simulink model "SingleTrack"  (R2019b)
settings: Solver=ode1  StartTime=0  StopTime=250  FixedStep=1.0000000000000000e-003  RelTol=1e-3
InitFcn:
  | sampleTime = str2double(get_param(bdroot, 'FixedStep'));
undefined symbols (not defined in the file or in its folder): AccPedalPos, BrakePedalPos, BrakeSwitch, DiscIntNeverNeededParam, DYNA4, EngSpd, IgnitionSwitch, InitialGear, InitialSpeed, IntendedEngTrq, LeftIndicator, MainBrakePress, MaxGear, MDL, MinGear, RefAcc, RefLane, RefLatPos, RefPath, RefPathCurv, RefSpd, RefSpdPreview, RefSpdRetrospect, RightIndicator, SteeringWheelAng, SteeringWheelTrq, UserDefinedRefValue, vm_const
libraries: UtilitiesLibrary x31, simulink x18, WheelSystemModules x13, LongitudinalControllerModules x13, LateralControllerModules x7, AnimationBusselectorModules x5, EnvironmentModules x5, BasicEngineControlModules x5, MiscellaneousControlModules x5, Animation3Modules x4, AuxiliariesModules x4, ReducedTireModules x4
(part 6 of 32)

== system SingleTrack/Vehicle/Engine ==
  fromCTRL : Inport
  fromEnvironment : Inport  Port=2
  fromChassis : Inport  Port=3
  fromDrivetrain : Inport  Port=4
  fromElectricalSystem : Inport  Port=5
  DYNA4 Trace Marker : UtilitiesLibrary/DYNA4 Trace Marker  Tag=DYNA4_TRACE_MARKER  SettingType=Standard  PrefixModelBlockID=on  PrefixRootSignalName=off  NamePattern='$(modelBlockID).$(rootSignalName)'
  DynaComponentInfo : Subsystem  Tag=DynaComponentInfo
      mask init:
      | data= get_param(gcb, 'UserData');
      settings: OpenFcn=DYNA4.ModelHandling.Component.ShowEditComponentInformationDialog(gcb);
      mask Display: disp(['Type = ', data.type, '\nGroup = ', data.group, '\nName = ', data.name ])
  EngineControlUnit : Subsystem  Tag=COMPONENT_ENGINE
  EngineOutputs : Subsystem  Tag=TESIS DYNAware Interface Block  mask{NeedsUpdate=off, SignalInfo=|}
      mask SignalInfo=|
      | {
      |   "Version": "4.6",
      |   "MuxedOutputBusName": "Engine",
      |   "MuxedInputBusName": "",
      |   "MuxedInputSelected": false,
      |   "MuxedOutputSelected": true,
      |   "SignalData": [
      |     {
      |       "initialValue": "0.0",
      |       "name": "EnginePhysics",
      |       "comment": "",
      |       "minString": "",
      |       "maxString": "",
      |       "width": -1,
      |       "dataType": 0,
      |       "signalType": 1,
      |       "createSignal": false,
      |       "outputName": "EnginePhysics",
      |       "generateSignalAccessBlock": false,
      |       "accessId": "$(parentId).$(blockName).$(outputName)"
      |     },
      |     {
      |       "initialValue": "0.0",
      |       "name": "EngineControlUnit",
      |       "comment": "",
      |       "minString": "",
      |       "maxString": "",
      |       "width": -1,
      |       "dataType": 0,
      |       "signalType": 1,
      |       "createSignal": false,
      |       "outputName": "EngineControlUnit",
      |       "generateSignalAccessBlock": false,
      |       "accessId": "$(parentId).$(blockName).$(outputName)"
      |     }
      |   ]
      | }
      mask prompts: NeedsUpdate "Specify, if subsystem content needs to be updated"; SignalInfo "Signal Info (json)"
      mask help: DYNA4 Interface Block Version 4.6
      mask init:
      | blockName = get_param(gcbh, 'Name');
      | parentId = DYNA4.ModelHandling.AccessID.getFromHierarchy(gcbh);
      | TD.InterfaceBlock.ModelCallbacks.GenerateContent(gcb);
      settings: DeleteFcn=TD.InterfaceBlock.ModelCallbacks.CloseGUI( gcbh );  NameChangeFcn=TD.InterfaceBlock.ModelCallbacks.BlockRenamedHandler(gcbh);  OpenFcn=TD.InterfaceBlock.ModelCallbacks.OpenGUI( gcbh );  CloseFcn=TD.InterfaceBlock.ModelCallbacks.CloseGUI( gcbh );
      mask Display:
      | image('InterfaceBlock.png','center');
      | port_label('input',1, 'EnginePhysics');
      | port_label('input',2, 'EngineControlUnit');
      | port_label('output',1, 'Engine');
  EnginePhysics : Subsystem  Tag=COMPONENT_ENGINE
  Engine : Outport  VectorParamsAs1DForOutWhenUnconnected=off
  wires:
  fromChassis/1 -> EnginePhysics/4(fromChassis), EngineControlUnit/4(fromChassis)
  EngineControlUnit/1(EngineControlUnit) -> EngineOutputs/2(EngineControlUnit___UNIQUE_1), EnginePhysics/1(fromEngineControlUnit)
  fromCTRL/1 -> EnginePhysics/2(fromCTRL), EngineControlUnit/2(fromCTRL)
  fromElectricalSystem/1 -> EnginePhysics/6(fromElectricalSystem), EngineControlUnit/6(fromElectricalSystem)
  fromEnvironment/1 -> EnginePhysics/3(fromEnvironment), EngineControlUnit/3(fromEnvironment)
  EngineOutputs/1(Engine___UNIQUE_1) -> Engine/1, DYNA4 Trace Marker/1
  fromDrivetrain/1 -> EnginePhysics/5(fromDrivetrain), EngineControlUnit/5(fromDrivetrain)
  EnginePhysics/1(EnginePhysics) -> EngineOutputs/1(EnginePhysics___UNIQUE_1), EngineControlUnit/1(fromEnginePhysics)

== system SingleTrack/Vehicle/VehicleOutput ==
  Auxiliaries___UNIQUE_1 : Inport  Description=|
      | <name>Auxiliaries</name>
      | <comment></comment>
  BrakeSystem___UNIQUE_1 : Inport  Description=|  Port=2
      | <name>BrakeSystem</name>
      | <comment></comment>
  Chassis___UNIQUE_1 : Inport  Description=|  Port=3
      | <name>Chassis</name>
      | <comment></comment>
  Drivetrain___UNIQUE_1 : Inport  Description=|  Port=4
      | <name>Drivetrain</name>
      | <comment></comment>
  ElectricalSystem___UNIQUE_1 : Inport  Description=|  Port=5
      | <name>ElectricalSystem</name>
      | <comment></comment>
  Engine___UNIQUE_1 : Inport  Description=|  Port=6
      | <name>Engine</name>
      | <comment></comment>
  WheelSystem___UNIQUE_1 : Inport  Description=|  Port=7
      | <name>WheelSystem</name>
      | <comment></comment>
  CoolingSystem___UNIQUE_1 : Inport  Description=|  Port=8
      | <name>CoolingSystem</name>
      | <comment></comment>
  VehicleRoadInfo___UNIQUE_1 : Inport  Description=|  Port=9
      | <name>VehicleRoadInfo</name>
      | <comment></comment>
  VehicleDriverInfo___UNIQUE_1 : Inport  Description=|  Port=10
      | <name>VehicleDriverInfo</name>
      | <comment></comment>
  __TDO__Vehicle : BusCreator  Inputs=10
  Vehicle___UNIQUE_1 : Outport  Description=|  VectorParamsAs1DForOutWhenUnconnected=off
      | <name>Auxiliaries</name>
      | <comment></comment>
  wires:
  __TDO__Vehicle/1 -> Vehicle___UNIQUE_1/1  "Vehicle"
  VehicleDriverInfo___UNIQUE_1/1 -> __TDO__Vehicle/10  "VehicleDriverInfo"
  VehicleRoadInfo___UNIQUE_1/1 -> __TDO__Vehicle/9  "VehicleRoadInfo"
  CoolingSystem___UNIQUE_1/1 -> __TDO__Vehicle/8  "CoolingSystem"
  WheelSystem___UNIQUE_1/1 -> __TDO__Vehicle/7  "WheelSystem"
  Engine___UNIQUE_1/1 -> __TDO__Vehicle/6  "Engine"
  ElectricalSystem___UNIQUE_1/1 -> __TDO__Vehicle/5  "ElectricalSystem"
  Drivetrain___UNIQUE_1/1 -> __TDO__Vehicle/4  "Drivetrain"
  Chassis___UNIQUE_1/1 -> __TDO__Vehicle/3  "Chassis"
  BrakeSystem___UNIQUE_1/1 -> __TDO__Vehicle/2  "BrakeSystem"
  Auxiliaries___UNIQUE_1/1 -> __TDO__Vehicle/1  "Auxiliaries"

== system SingleTrack/Vehicle/VehicleRoadInfo ==
  fromCTRL : Inport
  fromChassis : Inport  Port=2
  AdditionalRoadElevationAndRoadSlopes : Subsystem
  Demux : Demux  Outputs=3
  Demux1 : Demux  Outputs=2
  Demux2 : Demux  Outputs=2
  DynaComponentInfo : Subsystem  Tag=DynaComponentInfo
      mask init:
      | data = get_param(gcb, 'UserData');
      settings: OpenFcn=DYNA4.ModelHandling.Component.ShowEditComponentInformationDialog(gcb);
      mask Display: disp(['Type = ', data.type, '\nGroup = ', data.group, '\nName = ', data.name ])
  InputFromCTRL : Subsystem  Tag=TESIS DYNAware Interface Block  mask{NeedsUpdate=off, SignalInfo=|}
      mask SignalInfo=|
      | {
      |   "Version": "4.6",
      |   "MuxedOutputBusName": "output",
      |   "MuxedInputBusName": "fromCTRL",
      |   "MuxedInputSelected": true,
      |   "MuxedOutputSelected": false,
      |   "SignalData": [
      |     {
      |       "initialValue": "0.0",
      |       "name": "CTRL.AdditionalRoadElevation.FrontLeftAddRoadElev[m]",
      |       "comment": "",
      |       "minString": "",
      |       "maxString": "",
      |       "width": 1,
      |       "dataType": 0,
      |       "signalType": 0,
      |       "createSignal": false,
      |       "outputName": "FrontLeftAddRoadElev[m]",
      |       "generateSignalAccessBlock": false,
      |       "accessId": "$(parentId).$(blockName).$(outputName)"
      |     },
      |     {
      |       "initialValue": "0.0",
      |       "name": "CTRL.AdditionalRoadElevation.FrontRightAddRoadElev[m]",
      |       "comment": "",
      |       "minString": "",
      |       "maxString": "",
      |       "width": 1,
      |       "dataType": 0,
      |       "signalType": 0,
      |       "createSignal": false,
      |       "outputName": "FrontRightAddRoadElev[m]",
      |       "generateSignalAccessBlock": false,
      |       "accessId": "$(parentId).$(blockName).$(outputName)"
      |     },
      |     {
      |       "initialValue": "0.0",
      |       "name": "CTRL.AdditionalRoadElevation.AddLongRoadSlope[-]",
      |       "comment": "",
      |       "minString": "",
      |       "maxString": "",
      |       "width": 1,
      |       "dataType": 0,
      |       "signalType": 0,
      |       "createSignal": false,
      |       "outputName": "AddLongRoadSlope[-]",
      |       "generateSignalAccessBlock": false,
      |       "accessId": "$(parentId).$(blockName).$(outputName)"
      |     },
      |     {
      |       "initialValue": "0.0",
      |       "name": "CTRL.AdditionalRoadElevation.AddLatRoadSlope[-]",
      |       "comment": "",
      |       "minString": "",
      |       "maxString": "",
      |       "width": 1,
      |       "dataType": 0,
      |       "signalType": 0,
      |       "createSignal": false,
      |       "outputName": "AddLatRoadSlope[-]",
      |       "generateSignalAccessBlock": false,
      |       "accessId": "$(parentId).$(blockName).$(outputName)"
      |     },
      |     {
      |       "initialValue": "0.0",
      |       "name": "CTRL.AdditionalRoadElevation.LocalRoadSysSwitch[0;1]",
      |       "comment": "",
      |       "minString": "",
      |       "maxString": "",
      |       "width": 1,
      |       "dataType": 0,
      |       "signalType": 0,
      |       "createSignal": false,
      |       "outputName": "LocalRoadSysSwitch[0;1]",
      |       "generateSignalAccessBlock": false,
      |       "accessId": "$(parentId).$(blockName).$(outputName)"
      |     }
      |   ]
      | }
      mask prompts: NeedsUpdate "Specify, if subsystem content needs to be updated"; SignalInfo "Signal Info (json)"
      mask help: DYNA4 Interface Block Version 4.6
      mask init:
      | blockName = get_param(gcbh, 'Name');
      | parentId = DYNA4.ModelHandling.AccessID.getFromHierarchy(gcbh);
      | TD.InterfaceBlock.ModelCallbacks.GenerateContent(gcb);
      settings: DeleteFcn=TD.InterfaceBlock.ModelCallbacks.CloseGUI( gcbh );  NameChangeFcn=TD.InterfaceBlock.ModelCallbacks.BlockRenamedHandler(gcbh);  OpenFcn=TD.InterfaceBlock.ModelCallbacks.OpenGUI( gcbh );  CloseFcn=TD.InterfaceBlock.ModelCallbacks.CloseGUI( gcbh );
      mask Display:
      | image('InterfaceBlock.png','center');
      | port_label('input',1, 'fromCTRL');
      | port_label('output',1, 'FrontLeftAddRoadElev[m]');
      | port_label('output',2, 'FrontRightAddRoadElev[m]');
      | port_label('output',3, 'AddLongRoadSlope[-]');
      | port_label('output',4, 'AddLatRoadSlope[-]');
      | port_label('output',5, 'LocalRoadSysSwitch[0;1]');
  InputFromChassis : Subsystem  Tag=TESIS DYNAware Interface Block  mask{NeedsUpdate=off, SignalInfo=|}
      mask SignalInfo=|
      | {
      |   "Version": "4.6",
      |   "MuxedOutputBusName": "output",
      |   "MuxedInputBusName": "fromChassis",
      |   "MuxedInputSelected": true,
      |   "MuxedOutputSelected": false,
      |   "SignalData": [
      |     {
      |       "initialValue": "0.0",
      |       "name": "VehicleBody.Pos(WorldSys)[m]",
      |       "comment": "",
      |       "minString": "",
      |       "maxString": "",
      |       "width": 3,
      |       "dataType": 0,
      |       "signalType": 0,
      |       "createSignal": false,
      |       "outputName": "Pos(WorldSys)[m]",
      |       "generateSignalAccessBlock": false,
      |       "accessId": "$(parentId).$(blockName).$(outputName)"
      |     },
      |     {
      |       "initialValue": "0.0",
      |       "name": "VehicleBody.YawAng[rad]",
      |       "comment": "",
      |       "minString": "",
      |       "maxString": "",
      |       "width": 1,
      |       "dataType": 0,
      |       "signalType": 0,
      |       "createSignal": false,
      |       "outputName": "YawAng[rad]",
      |       "generateSignalAccessBlock": false,
      |       "accessId": "$(parentId).$(blockName).$(outputName)"
      |     }
      |   ]
      | }
      mask prompts: NeedsUpdate "Specify, if subsystem content needs to be updated"; SignalInfo "Signal Info (json)"
      mask help: DYNA4 Interface Block Version 4.6
      mask init:
      | blockName = get_param(gcbh, 'Name');
      | parentId = DYNA4.ModelHandling.AccessID.getFromHierarchy(gcbh);
      | TD.InterfaceBlock.ModelCallbacks.GenerateContent(gcb);
      settings: DeleteFcn=TD.InterfaceBlock.ModelCallbacks.CloseGUI( gcbh );  NameChangeFcn=TD.InterfaceBlock.ModelCallbacks.BlockRenamedHandler(gcbh);  OpenFcn=TD.InterfaceBlock.ModelCallbacks.OpenGUI( gcbh );  CloseFcn=TD.InterfaceBlock.ModelCallbacks.CloseGUI( gcbh );
      mask Display:
      | image('InterfaceBlock.png','center');
      | port_label('input',1, 'fromChassis');
      | port_label('output',1, 'Pos(WorldSys)[m]');
      | port_label('output',2, 'YawAng[rad]');
  Road Information : RoadModules/Road Information  RoadQueryType=X, Y (WorldSystem)  RoadQueryNumber=1  ODR_ALL_FLAGS=off  ODR_TRACKID=on  ODR_LANEID=on  ODR_XY=off  ODR_Z=on  ODR_S_ROAD=on  ODR_Q_ROAD=on  ODR_Q_PATH=off  ODR_QMINMAX_ROAD=off  ODR_QMINMAX_PATH=off  ODR_XY_REF=off  ODR_GEO_COORDINATES=off  ODR_ANGLE_ROAD=on  ODR_ANGLE_PATH=off  ODR_CURVATURE_ROAD=on  ODR_CURVATURE_PATH=on  ODR_TXTY_ROAD=on  ODR_PITCHROLL_ROAD=off  ODR_SQSLOPE_ROAD=on  ODR_MATERIAL=on  ODR_LATERAL_INFO=off  ODR_NEXT_DRIVEABLE_LANEID=off  ODR_ROAD_MARKS=off  ODR_VMAX=off  ODR_ROAD_SIGNS=off  ODR_ROUTE=off  ODR_JUNCTION=off  ODR_ROAD_LANE_LIST=off  ODR_LENGTH_CLOSED=on  EnableSeparateRoute=off  RoutePointsTrackIDs=MDL.Traffic.TrafficObjects.Traffic.Route{1}.RoutePointsTrackIDs.v  RoutePointsSCoordOnTrack=MDL.Traffic.TrafficObjects.Traffic.Route{1}.RoutePointsSCoordOnTrack.v  sample_time=-1
  Selector1 : Selector  InputPortWidth=3  IndexOptions=Index vector (dialog)  Indices=[1 2]  OutputSizes=1
  Selector2 : Selector  InputPortWidth=6  IndexOptions=Index vector (dialog)  Indices=[1 2]  OutputSizes=1
  Sum : Sum  Inputs=|++
  Sum1 : Sum  Inputs=|++
  Sum3 : Sum  Inputs=|++
  Terminator : Terminator
  TraceMarker : UtilitiesLibrary/DYNA4 Trace Marker  Tag=DYNA4_TRACE_MARKER  SettingType=Standard  PrefixModelBlockID=on  PrefixRootSignalName=off  NamePattern='$(modelBlockID).$(rootSignalName)'
  VehicleRoadInfoOutput : Subsystem  Tag=TESIS DYNAware Interface Block  mask{NeedsUpdate=off, SignalInfo=|}
      mask SignalInfo=|
      | {
      |   "Version": "4.6",
      |   "MuxedOutputBusName": "VehicleRoadInfo",
      |   "MuxedInputBusName": "input",
      |   "MuxedInputSelected": false,
      |   "MuxedOutputSelected": true,
      |   "SignalData": [
      |     {
      |       "initialValue": "0.0",
      |       "name": "TrackID[-]",
      |       "comment": "",
      |       "minString": "",
      |       "maxString": "",
      |       "width": 1,
      |       "dataType": 0,
      |       "signalType": 0,
      |       "createSignal": false,
      |       "outputName": "TrackID[-]",
      |       "generateSignalAccessBlock": false,
      |       "accessId": "$(parentId).$(blockName).$(outputName)"
      |     },
      |     {
      |       "initialValue": "0.0",
      |       "name": "LaneID[-]",
      |       "comment": "",
      |       "minString": "",
      |       "maxString": "",
      |       "width": 1,
      |       "dataType": 0,
      |       "signalType": 0,
      |       "createSignal": false,
      |       "outputName": "LaneID[-]",
      |       "generateSignalAccessBlock": false,
      |       "accessId": "$(parentId).$(blockName).$(outputName)"
      |     },
      |     {
      |       "initialValue": "0.0",
      |       "name": "RoadZ[m]",
      |       "comment": "",
      |       "minString": "",
      |       "maxString": "",
      |       "width": 1,
      |       "dataType": 0,
      |       "signalType": 0,
      |       "createSignal": false,
      |       "outputName": "RoadZ[m]",
      |       "generateSignalAccessBlock": false,
      |       "accessId": "$(parentId).$(blockName).$(outputName)"
      |     },
      |     {
      |       "initialValue": "0.0",
      |       "name": "RoadS[m]",
      |       "comment": "",
      |       "minString": "",
      |       "maxString": "",
      |       "width": 1,
      |       "dataType": 0,
      |       "signalType": 0,
      |       "createSignal": false,
      |       "outputName": "RoadS[m]",
      |       "generateSignalAccessBlock": false,
      |       "accessId": "$(parentId).$(blockName).$(outputName)"
      |     },
      |     {
      |       "initialValue": "0.0",
      |       "name": "RoadQ[m]",
      |       "comment": "",
      |       "minString": "",
      |       "maxString": "",
      |       "width": 1,
      |       "dataType": 0,
      |       "signalType": 0,
      |       "createSignal": false,
      |       "outputName": "RoadQ[m]",
      |       "generateSignalAccessBlock": false,
      |       "accessId": "$(parentId).$(blockName).$(outputName)"
      |     },
      |     {
      |       "initialValue": "0.0",
      |       "name": "RoadAngle[rad]",
      |       "comment": "",
      |       "minString": "",
      |       "maxString": "",
      |       "width": 1,
      |       "dataType": 0,
      |       "signalType": 0,
      |       "createSignal": false,
      |       "outputName": "RoadAngle[rad]",
      |       "generateSignalAccessBlock": false,
      |       "accessId": "$(parentId).$(blockName).$(outputName)"
      |     },
      |     {
      |       "initialValue": "0.0",
      |       "name": "RoadCurvature[1/m]",
      |       "comment": "",
      |       "minString": "",
      |       "maxString": "",
      |       "width": 1,
      |       "dataType": 0,
      |       "signalType": 0,
      |       "createSignal": false,
      |       "outputName": "RoadCurvature[1/m]",
      |       "generateSignalAccessBlock": false,
      |       "accessId": "$(parentId).$(blockName).$(outputName)"
      |     },
      |     {
      |       "initialValue": "0.0",
      |       "name": "LaneCurvature[1/m]",
      |       "comment": "",
      |       "minString": "",
      |       "maxString": "",
      |       "width": 1,
      |       "dataType": 0,
      |       "signalType": 0,
      |       "createSignal": false,
      |       "outputName": "LaneCurvature[1/m]",
      |       "generateSignalAccessBlock": false,
      |       "accessId": "$(parentId).$(blockName).$(outputName)"
      |     },
      |     {
      |       "initialValue": "0.0",
      |       "name": "RoadTangentXY[-]",
      |       "comment": "",
      |       "minString": "",
      |       "maxString": "",
      |       "width": 2,
      |       "dataType": 0,
      |       "signalType": 0,
      |       "createSignal": false,
      |       "outputName": "RoadTangentXY[-]",
      |       "generateSignalAccessBlock": false,
      |       "accessId": "$(parentId).$(blockName).$(outputName)"
      |     },
      |     {
      |       "initialValue": "0.0",
      |       "name": "RoadSlopeLong[-]",
      |       "comment": "",
      |       "minString": "",
      |       "maxString": "",
      |       "width": 1,
      |       "dataType": 0,
      |       "signalType": 0,
      |       "createSignal": false,
      |       "outputName": "RoadSlopeLong[-]",
      |       "generateSignalAccessBlock": false,
      |       "accessId": "$(parentId).$(blockName).$(outputName)"
      |     },
      |     {
      |       "initialValue": "0.0",
      |       "name": "RoadSlopeLat[-]",
      |       "comment": "",
      |       "minString": "",
      |       "maxString": "",
      |       "width": 1,
      |       "dataType": 0,
      |       "signalType": 0,
      |       "createSignal": false,
      |       "outputName": "RoadSlopeLat[-]",
      |       "generateSignalAccessBlock": false,
      |       "accessId": "$(parentId).$(blockName).$(outputName)"
      |     },
      |     {
      |       "initialValue": "0.0",
      |       "name": "RoadFriction[-]",
      |       "comment": "",
      |       "minString": "",
      |       "maxString": "",
      |       "width": 1,
      |       "dataType": 0,
      |       "signalType": 0,
      |       "createSignal": false,
      |       "outputName": "RoadFriction[-]",
      |       "generateSignalAccessBlock": false,
      |       "accessId": "$(parentId).$(blockName).$(outputName)"
      |     },
      |     {
      |       "initialValue": "0.0",
      |       "name": "RoadSurfaceType[-]",
      |       "comment": "",
      |       "minString": "",
      |       "maxString": "",
      |       "width": 1,
      |       "dataType": 0,
      |       "signalType": 0,
      |       "createSignal": false,
      |       "outputName": "RoadSurfaceType[-]",
      |       "generateSignalAccessBlock": false,
      |       "accessId": "$(parentId).$(blockName).$(outputName)"
      |     },
      |     {
      |       "initialValue": "0.0",
      |       "name": "RoadRoughness[-]",
      |       "comment": "",
      |       "minString": "",
      |       "maxString": "",
      |       "width": 1,
      |       "dataType": 0,
      |       "signalType": 0,
      |       "createSignal": false,
      |       "outputName": "RoadRoughness[-]",
      |       "generateSignalAccessBlock": false,
      |       "accessId": "$(parentId).$(blockName).$(outputName)"
      |     },
      |     {
      |       "initialValue": "0.0",
      |       "name": "RouteLength[m]",
      |       "comment": "",
      |       "minString": "",
      |       "maxString": "",
      |       "width": 1,
      |       "dataType": 0,
      |       "signalType": 0,
      |       "createSignal": false,
      |       "outputName": "RouteLength[m]",
      |       "generateSignalAccessBlock": false,
      |       "accessId": "$(parentId).$(blockName).$(outputName)"
      |     },
      |     {
      |       "initialValue": "0.0",
      |       "name": "RouteClosed[-]",
      |       "comment": "",
      |       "minString": "",
      |       "maxString": "",
      |       "width": 1,
      |       "dataType": 0,
      |       "signalType": 0,
      |       "createSignal": false,
      |       "outputName": "RouteClosed[-]",
      |       "generateSignalAccessBlock": false,
      |       "accessId": "$(parentId).$(blockName).$(outputName)"
      |     }
      |   ]
      | }
      mask prompts: NeedsUpdate "Specify, if subsystem content needs to be updated"; SignalInfo "Signal Info (json)"
      mask help: DYNA4 Interface Block Version 4.6
      mask init:
      | blockName = get_param(gcbh, 'Name');
      | parentId = DYNA4.ModelHandling.AccessID.getFromHierarchy(gcbh);
      | TD.InterfaceBlock.ModelCallbacks.GenerateContent(gcb);
      settings: DeleteFcn=TD.InterfaceBlock.ModelCallbacks.CloseGUI( gcbh );  NameChangeFcn=TD.InterfaceBlock.ModelCallbacks.BlockRenamedHandler(gcbh);  OpenFcn=TD.InterfaceBlock.ModelCallbacks.OpenGUI( gcbh );  CloseFcn=TD.InterfaceBlock.ModelCallbacks.CloseGUI( gcbh );
      mask Display:
      | image('InterfaceBlock.png','center');
      | port_label('input',1, 'TrackID[-]');
      | port_label('input',2, 'LaneID[-]');
      | port_label('input',3, 'RoadZ[m]');
      | port_label('input',4, 'RoadS[m]');
      | port_label('input',5, 'RoadQ[m]');
      | port_label('input',6, 'RoadAngle[rad]');
      | port_label('input',7, 'RoadCurvature[1/m]');
      | port_label('input',8, 'LaneCurvature[1/m]');
      | port_label('input',9, 'RoadTangentXY[-]');
      | port_label('input',10, 'RoadSlopeLong[-]');
      | port_label('input',11, 'RoadSlopeLat[-]');
      | port_label('input',12, 'RoadFriction[-]');
      | port_label('input',13, 'RoadSurfaceType[-]');
      | port_label('input',14, 'RoadRoughness[-]');
      | port_label('input',15, 'RouteLength[m]');
      | port_label('input',16, 'RouteClosed[-]');
      | port_label('output',1, 'VehicleRoadInfo');
  VehicleRoadInfo : Outport  VectorParamsAs1DForOutWhenUnconnected=off
  tag scope: VehicleRoadInfo=global
  wires:
  InputFromChassis/2(YawAng[rad]___UNIQUE_1) -> AdditionalRoadElevationAndRoadSlopes/1(YawAng[rad])
  InputFromChassis/1(Pos(WorldSys)[m]___UNIQUE_1) -> Selector1/1
  AdditionalRoadElevationAndRoadSlopes/3(AddLatRoadSlope[-]) -> Sum1/2
  AdditionalRoadElevationAndRoadSlopes/2(AddLongRoadSlope[-]) -> Sum/2
  AdditionalRoadElevationAndRoadSlopes/1(FrontAdditionalRoadElev[m]) -> Sum3/2
  InputFromCTRL/5(LocalRoadSysSwitch[0;1]___UNIQUE_1) -> AdditionalRoadElevationAndRoadSlopes/6(LocalRoadSysSwitch[0;1])
  InputFromCTRL/4(AddLatRoadSlope[-]___UNIQUE_1) -> AdditionalRoadElevationAndRoadSlopes/5(AddLatRoadSlopeIn[-])
  InputFromCTRL/3(AddLongRoadSlope[-]___UNIQUE_1) -> AdditionalRoadElevationAndRoadSlopes/4(AddLongRoadSlopeIn[-])
  InputFromCTRL/2(FrontRightAddRoadElev[m]___UNIQUE_1) -> AdditionalRoadElevationAndRoadSlopes/3(FrontRightAddRoadElev[m])
  InputFromCTRL/1(FrontLeftAddRoadElev[m]___UNIQUE_1) -> AdditionalRoadElevationAndRoadSlopes/2(FrontLeftAddRoadElev[m])
  Sum3/1 -> VehicleRoadInfoOutput/3(RoadZ[m]___UNIQUE_1)
  Road Information/3 -> Sum3/1
  Sum1/1 -> VehicleRoadInfoOutput/11(RoadSlopeLat[-]___UNIQUE_1)
  Demux1/2 -> Sum1/1
  Sum/1 -> VehicleRoadInfoOutput/10(RoadSlopeLong[-]___UNIQUE_1)
  Demux1/1 -> Sum/1
  fromCTRL/1 -> InputFromCTRL/1(fromCTRL)
  Road Information/12 -> Selector2/1
  Road Information/11 -> Demux/1
  Road Information/10 -> Demux1/1
  Road Information/9 -> VehicleRoadInfoOutput/9(RoadTangentXY[-]___UNIQUE_1)
  Road Information/8 -> VehicleRoadInfoOutput/8(LaneCurvature[1/m]___UNIQUE_1)
  Road Information/7 -> VehicleRoadInfoOutput/7(RoadCurvature[1/m]___UNIQUE_1)
  Selector2/1 -> Demux2/1
  Demux2/2 -> VehicleRoadInfoOutput/16(RouteClosed[-]___UNIQUE_1)
  Demux2/1 -> VehicleRoadInfoOutput/15(RouteLength[m]___UNIQUE_1)
  Demux/3 -> VehicleRoadInfoOutput/14(RoadRoughness[-]___UNIQUE_1)
  Demux/2 -> VehicleRoadInfoOutput/13(RoadSurfaceType[-]___UNIQUE_1)
  Demux/1 -> VehicleRoadInfoOutput/12(RoadFriction[-]___UNIQUE_1)
  Road Information/6 -> VehicleRoadInfoOutput/6(RoadAngle[rad]___UNIQUE_1)
  Road Information/5 -> VehicleRoadInfoOutput/5(RoadQ[m]___UNIQUE_1)
  Road Information/4 -> VehicleRoadInfoOutput/4(RoadS[m]___UNIQUE_1)
  Road Information/2 -> VehicleRoadInfoOutput/2(LaneID[-]___UNIQUE_1)
  Road Information/1 -> VehicleRoadInfoOutput/1(TrackID[-]___UNIQUE_1)
  Selector1/1 -> Road Information/2
  fromChassis/1 -> InputFromChassis/1(fromChassis)
  VehicleRoadInfoOutput/1(VehicleRoadInfo___UNIQUE_1) -> TraceMarker/1, [VehicleRoadInfo], VehicleRoadInfo/1
  [IRoadInterface] -> Road Information/1
  [VehicleRoadInfo] -> Terminator/1

== system SingleTrack/Vehicle/WheelSystem ==
  fromCTRL : Inport
  fromBrakeSystem : Inport  Port=2
  fromChassis : Inport  Port=3
  fromDrivetrain : Inport  Port=4
  DynaComponentInfo : Subsystem  Tag=DynaComponentInfo
      mask init:
      | data= get_param(gcb, 'UserData');
      settings: OpenFcn=DYNA4.ModelHandling.Component.ShowEditComponentInformationDialog(gcb);
      mask Display: disp(['Type = ', data.type, '\nGroup = ', data.group, '\nName = ', data.name])
  FrontLeftWheelSystem : Subsystem
  FrontRightWheelSystem : Subsystem
  RearLeftWheelSystem : Subsystem
  RearRightWheelSystem : Subsystem
  WheelSystemInputs : WheelSystemModules/WheelSystemInputs  SystemSampleTime=-1  Latency=0  AutoFrameSizeCalculation=off
  WheelSystemOutputs : Subsystem
  WheelSystem : Outport  VectorParamsAs1DForOutWhenUnconnected=off
  wires:
  WheelSystemInputs/12 -> RearLeftWheelSystem/4(fromBrakeSystem)
  RearRightWheelSystem/3(WheelStates) -> WheelSystemOutputs/12(RearRightWheelStates)
  RearRightWheelSystem/2(TireStates) -> WheelSystemOutputs/11(RearRightTireStates)
  RearRightWheelSystem/1(InnerTireStates) -> WheelSystemOutputs/10(RearRightInnerTireStates)
  RearLeftWheelSystem/3(WheelStates) -> WheelSystemOutputs/9(RearLeftWheelStates)
  RearLeftWheelSystem/2(TireStates) -> WheelSystemOutputs/8(RearLeftTireStates)
  RearLeftWheelSystem/1(InnerTireStates) -> WheelSystemOutputs/7(RearLeftInnerTireStates)
  FrontRightWheelSystem/3(WheelStates) -> WheelSystemOutputs/6(FrontRightWheelStates)
  FrontRightWheelSystem/2(TireStates) -> WheelSystemOutputs/5(FrontRightTireStates)
  FrontRightWheelSystem/1(InnerTireStates) -> WheelSystemOutputs/4(FrontRightInnerTireStates)
  WheelSystemInputs/4 -> FrontLeftWheelSystem/4(fromBrakeSystem)
  WheelSystemInputs/3 -> FrontLeftWheelSystem/3(fromDrivetrain)
  WheelSystemInputs/2 -> FrontLeftWheelSystem/2(fromCTRL)
  WheelSystemInputs/1 -> FrontLeftWheelSystem/1(fromChassis)
  WheelSystemInputs/16 -> RearRightWheelSystem/4(fromBrakeSystem)
  WheelSystemInputs/15 -> RearRightWheelSystem/3(fromDrivetrain)
  WheelSystemInputs/14 -> RearRightWheelSystem/2(fromCTRL)
  WheelSystemInputs/13 -> RearRightWheelSystem/1(fromChassis)
  WheelSystemInputs/11 -> RearLeftWheelSystem/3(fromDrivetrain)
  WheelSystemInputs/10 -> RearLeftWheelSystem/2(fromCTRL)
  WheelSystemInputs/9 -> RearLeftWheelSystem/1(fromChassis)
  WheelSystemInputs/8 -> FrontRightWheelSystem/4(fromBrakeSystem)
  WheelSystemInputs/7 -> FrontRightWheelSystem/3(fromDrivetrain)
  WheelSystemInputs/6 -> FrontRightWheelSystem/2(fromCTRL)
  WheelSystemInputs/5 -> FrontRightWheelSystem/1(fromChassis)
  FrontLeftWheelSystem/3(WheelStates) -> WheelSystemOutputs/3(FrontLeftWheelStates)
  FrontLeftWheelSystem/2(TireStates) -> WheelSystemOutputs/2(FrontLeftTireStates)
  FrontLeftWheelSystem/1(InnerTireStates) -> WheelSystemOutputs/1(FrontLeftInnerTireStates)
  fromCTRL/1 -> WheelSystemInputs/4
  fromBrakeSystem/1 -> WheelSystemInputs/3
  fromChassis/1 -> WheelSystemInputs/2
  fromDrivetrain/1 -> WheelSystemInputs/1
  WheelSystemOutputs/1(WheelSystem) -> WheelSystem/1

== system SingleTrack/VehicleControl/DynaComponentInfo ==

== system SingleTrack/VehicleControl/InitialConditions ==
  fromCTRL : Inport
  InitialConditionsOutput : Subsystem  Tag=TESIS DYNAware Interface Block  mask{NeedsUpdate=off, SignalInfo=|}
      mask SignalInfo=|
      | {
      |   "Version": "4.6",
      |   "MuxedOutputBusName": "InitialConditions",
      |   "MuxedInputBusName": "fromCTRL",
      |   "MuxedInputSelected": false,
      |   "MuxedOutputSelected": true,
      |   "SignalData": [
      |     {
      |       "initialValue": "0.0",
      |       "name": "InitialPositionX(WorldSys)[m]",
      |       "comment": "Initial x-position in world coordinates",
      |       "minString": "",
      |       "maxString": "",
      |       "width": 1,
      |       "dataType": 0,
      |       "signalType": 0,
      |       "createSignal": false,
      |       "outputName": "InitialPositionX(WorldSys)[m]",
      |       "generateSignalAccessBlock": false,
      |       "accessId": "$(parentId).$(blockName).$(outputName)"
      |     },
      |     {
      |       "initialValue": "0.0",
      |       "name": "InitialPositionY(WorldSys)[m]",
      |       "comment": "Initial y-position in world coordinates",
      |       "minString": "",
      |       "maxString": "",
      |       "width": 1,
      |       "dataType": 0,
      |       "signalType": 0,
      |       "createSignal": false,
      |       "outputName": "InitialPositionY(WorldSys)[m]",
      |       "generateSignalAccessBlock": false,
      |       "accessId": "$(parentId).$(blockName).$(outputName)"
      |     },
      |     {
      |       "initialValue": "0.0",
      |       "name": "InitialPositionZ(WorldSys)[m]",
      |       "comment": "Initial z-position in world coordinates",
      |       "minString": "",
      |       "maxString": "",
      |       "width": 1,
      |       "dataType": 0,
      |       "signalType": 0,
      |       "createSignal": false,
      |       "outputName": "InitialPositionZ(WorldSys)[m]",
      |       "generateSignalAccessBlock": false,
      |       "accessId": "$(parentId).$(blockName).$(outputName)"
      |     },
      |     {
      |       "initialValue": "0.0",
      |       "name": "InitialRoll[rad]",
      |       "comment": "Initial roll angle",
      |       "minString": "",
      |       "maxString": "",
      |       "width": 1,
      |       "dataType": 0,
      |       "signalType": 0,
      |       "createSignal": false,
      |       "outputName": "InitialRoll[rad]",
      |       "generateSignalAccessBlock": false,
      |       "accessId": "$(parentId).$(blockName).$(outputName)"
      |     },
      |     {
      |       "initialValue": "0.0",
      |       "name": "InitialPitch[rad]",
      |       "comment": "Initial pitch angle",
      |       "minString": "",
      |       "maxString": "",
      |       "width": 1,
      |       "dataType": 0,
      |       "signalType": 0,
      |       "createSignal": false,
      |       "outputName": "InitialPitch[rad]",
      |       "generateSignalAccessBlock": false,
      |       "accessId": "$(parentId).$(blockName).$(outputName)"
      |     },
      |     {
      |       "initialValue": "0.0",
      |       "name": "InitialYaw[rad]",
      |       "comment": "Initial yaw angle",
      |       "minString": "",
      |       "maxString": "",
      |       "width": 1,
      |       "dataType": 0,
      |       "signalType": 0,
      |       "createSignal": false,
      |       "outputName": "InitialYaw[rad]",
      |       "generateSignalAccessBlock": false,
      |       "accessId": "$(parentId).$(blockName).$(outputName)"
      |     }
      |   ]
      | }
      mask prompts: NeedsUpdate "Specify, if subsystem content needs to be updated"; SignalInfo "Signal Info (json)"
      mask help: DYNA4 Interface Block Version 4.6
      mask init:
      | blockName = get_param(gcbh, 'Name');
      | parentId = DYNA4.ModelHandling.AccessID.getFromHierarchy(gcbh);
      | TD.InterfaceBlock.ModelCallbacks.GenerateContent(gcb);
      settings: DeleteFcn=TD.InterfaceBlock.ModelCallbacks.CloseGUI( gcbh );  NameChangeFcn=TD.InterfaceBlock.ModelCallbacks.BlockRenamedHandler(gcbh);  OpenFcn=TD.InterfaceBlock.ModelCallbacks.OpenGUI( gcbh );  CloseFcn=TD.InterfaceBlock.ModelCallbacks.CloseGUI( gcbh );
      mask Display:
      | image('InterfaceBlock.png','center');
      | port_label('input',1, 'InitialPositionX(WorldSys)[m]');
      | port_label('input',2, 'InitialPositionY(WorldSys)[m]');
      | port_label('input',3, 'InitialPositionZ(WorldSys)[m]');
      | port_label('input',4, 'InitialRoll[rad]');
      | port_label('input',5, 'InitialPitch[rad]');
      | port_label('input',6, 'InitialYaw[rad]');
      | port_label('output',1, 'InitialConditions');
  InitialPosition : InitialConditionsModules/InitialPosition  DATA_NODE=MDL.VehicleControl.InitialPosition  InitialCoordinates=MDL.VehicleControl.InitialPosition.InitialCoordinates  InitialYawRotation=MDL.VehicleControl.InitialPosition.InitialYawRotation
  InitialConditions : Outport  VectorParamsAs1DForOutWhenUnconnected=off
  wires:
  InitialConditionsOutput/1(InitialConditions___UNIQUE_1) -> InitialConditions/1
  InitialPosition/1 -> InitialConditionsOutput/1(InitialPositionX(WorldSys)[m]___UNIQUE_1)
  InitialPosition/4 -> InitialConditionsOutput/4(InitialRoll[rad]___UNIQUE_1)
  InitialPosition/5 -> InitialConditionsOutput/5(InitialPitch[rad]___UNIQUE_1)
  InitialPosition/2 -> InitialConditionsOutput/2(InitialPositionY(WorldSys)[m]___UNIQUE_1)
  InitialPosition/6 -> InitialConditionsOutput/6(InitialYaw[rad]___UNIQUE_1)
  InitialPosition/3 -> InitialConditionsOutput/3(InitialPositionZ(WorldSys)[m]___UNIQUE_1)
  fromCTRL/1 -> InitialPosition/1

== system SingleTrack/VehicleControl/LateralControl ==
  SchedulerAbscissae : Inport
  CtrlSystemsAbscissae : Inport  Port=2
  PhaseTerminationVals : Inport  Port=3
  VehicleInfo : Inport  Port=4
  LatCTRL : Inport  Port=5
  ExtCtrlVariablesEnforced : Inport  Port=6
  ExtCtrlVals : Inport  Port=7
  Disabled LateralControl : Subsystem  VariantControl=DisabledLateralControl
  Enabled LateralControl : Subsystem  VariantControl=EnabledLateralControl
  LateralControl : Outport  VectorParamsAs1DForOutWhenUnconnected=off

== system SingleTrack/VehicleControl/LongitudinalControl ==
  SchedulerAbscissae : Inport
  CtrlSystemsAbscissae : Inport  Port=2
  PhaseTerminationVals : Inport  Port=3
  VehicleInfo : Inport  Port=4
  TrafficInfo : Inport  Port=5
  LongCTRL : Inport  Port=6
  ExtCtrlVariablesEnforced : Inport  Port=7
  ExtCtrlVals : Inport  Port=8
  ControlSystems : Subsystem
  ControlSystemsPreprocessor : Subsystem
  DynaSystemInfo : Subsystem  Tag=DynaSystemInfo
      mask init:
      | data = get_param(gcb, 'UserData');
      settings: OpenFcn=DYNA4.ModelHandling.System.ShowEditSystemInformationDialog(gcb);
      mask Display: disp(['Type = ', data.type, '\nName = ', data.name ])
  tsim : Selector  InputPortWidth=2  IndexOptions=Index vector (dialog)  Indices=1  OutputSizes=1
  LongitudinalControl : Outport  VectorParamsAs1DForOutWhenUnconnected=off
  wires:
  ControlSystemsPreprocessor/5(VehicleInfoSpeedControl) -> ControlSystems/6(VehicleInfoSpeedControl)
  ControlSystemsPreprocessor/1(Phase[-]) -> ControlSystems/2(Phase[-])
  ControlSystems/1(ControlOutputs) -> LongitudinalControl/1
  PhaseTerminationVals/1 -> ControlSystemsPreprocessor/2(PhaseTerminationVals)
  SchedulerAbscissae/1 -> tsim/1, ControlSystemsPreprocessor/1(SchedulerAbscissae)
  VehicleInfo/1 -> ControlSystemsPreprocessor/6(VehicleInfo)
  ControlSystemsPreprocessor/4(ControlInputs) -> ControlSystems/5(ControlInputs)
  ControlSystemsPreprocessor/3(SourceIdentifiers) -> ControlSystems/4(SourceIdentifiers)
  ControlSystemsPreprocessor/2(TaskIdentifiers) -> ControlSystems/3(TaskIdentifiers)
  CtrlSystemsAbscissae/1 -> ControlSystems/8(CtrlSystemsAbscissae), ControlSystemsPreprocessor/8(CtrlSystemsAbscissae)
  ExtCtrlVals/1 -> ControlSystemsPreprocessor/5(ExtCtrlVals)
  ExtCtrlVariablesEnforced/1 -> ControlSystemsPreprocessor/4(ExtCtrlVariablesEnforced)
  LongCTRL/1 -> ControlSystemsPreprocessor/3(LongCTRL)
  tsim/1 -> ControlSystems/1(SimulationTime[s])
  TrafficInfo/1 -> ControlSystemsPreprocessor/7(TrafficInfo)
  ControlSystems/2(SpeedControlParameters) -> ControlSystemsPreprocessor/9(SpeedControlParameters)
  ControlSystemsPreprocessor/6(UserDefinedSignals) -> ControlSystems/7(UserDefinedSignals)

== system SingleTrack/VehicleControl/Miscellaneous ==
  note: How to add user-defined miscellaneous signals to the model:
      |
      | 1. Open the block "UserDefinedControlOutput" by double-clicking on it.
      | 2. Edit the signals inside by renaming them and setting the unit. You can also add signals to the existing ones.
      | 3. Adjust the size of the demux-block on the left of the bus-creator so that all ports can be connected.
      | 4. Save the model to apply your changes.
  Abscissae : Inport
  BrakeHydraulicsControl : MiscellaneousControlModules/BrakeHydraulicsControl  DATA_NODE=MDL.VehicleControl.Miscellaneous.BrakeHydraulicsControl  Circuit1PumpSignal=MDL.VehicleControl.Miscellaneous.BrakeHydraulicsControl.Circuit1PumpSignal  Circuit1PressReliefValveCurr=MDL.VehicleControl.Miscellaneous.BrakeHydraulicsControl.Circuit1PressReliefValveCurr  Circuit1ReversingValveCurr=MDL.VehicleControl.Miscellaneous.BrakeHydraulicsControl.Circuit1ReversingValveCurr  Circuit2PumpSignal=MDL.VehicleControl.Miscellaneous.BrakeHydraulicsControl.Circuit2PumpSignal  Circuit2PressReliefValveCurr=MDL.VehicleControl.Miscellaneous.BrakeHydraulicsControl.Circuit2PressReliefValveCurr  Circuit2ReversingValveCurr=MDL.VehicleControl.Miscellaneous.BrakeHydraulicsControl.Circuit2ReversingValveCurr  FrontLeftInletValveCurr=MDL.VehicleControl.Miscellaneous.BrakeHydraulicsControl.FrontLeftInletValveCurr  FrontLeftOutletValveCurr=MDL.VehicleControl.Miscellaneous.BrakeHydraulicsControl.FrontLeftOutletValveCurr  FrontRightInletValveCurr=MDL.VehicleControl.Miscellaneous.BrakeHydraulicsControl.FrontRightInletValveCurr  FrontRightOutletValveCurr=MDL.VehicleControl.Miscellaneous.BrakeHydraulicsControl.FrontRightOutletValveCurr  RearLeftInletValveCurr=MDL.VehicleControl.Miscellaneous.BrakeHydraulicsControl.RearLeftInletValveCurr  RearLeftOutletValveCurr=MDL.VehicleControl.Miscellaneous.BrakeHydraulicsControl.RearLeftOutletValveCurr  RearRightInletValveCurr=MDL.VehicleControl.Miscellaneous.BrakeHydraulicsControl.RearRightInletValveCurr  RearRightOutletValveCurr=MDL.VehicleControl.Miscellaneous.BrakeHydraulicsControl.RearRightOutletValveCurr
  Demux : Demux  Outputs=2
  DynaSystemInfo : Subsystem  Tag=DynaSystemInfo
      mask init:
      | data = get_param(gcb, 'UserData');
      settings: OpenFcn=DYNA4.ModelHandling.System.ShowEditSystemInformationDialog(gcb);
      mask Display: disp(['Type = ', data.type, '\nName = ', data.name ])
  EngineControl : MiscellaneousControlModules/EngineControl  DATA_NODE=MDL.VehicleControl.Miscellaneous.EngineControl  RefEngSpd=MDL.VehicleControl.Miscellaneous.EngineControl.RefEngSpd  EngTrq=MDL.VehicleControl.Miscellaneous.EngineControl.EngTrq  FuelMass=MDL.VehicleControl.Miscellaneous.EngineControl.FuelMass  AftercoolerOutAirTemp=MDL.VehicleControl.Miscellaneous.EngineControl.AftercoolerOutAirTemp  IgnitionAng=MDL.VehicleControl.Miscellaneous.EngineControl.IgnitionAng  ThrottlePos=MDL.VehicleControl.Miscellaneous.EngineControl.ThrottlePos  ThrottleMassFlow=MDL.VehicleControl.Miscellaneous.EngineControl.ThrottleMassFlow  InjectionMassPre=MDL.VehicleControl.Miscellaneous.EngineControl.InjectionMassPre  InjectionMassMain=MDL.VehicleControl.Miscellaneous.EngineControl.InjectionMassMain  InjectionMassPost1=MDL.VehicleControl.Miscellaneous.EngineControl.InjectionMassPost1  InjectionMassPost2=MDL.VehicleControl.Miscellaneous.EngineControl.InjectionMassPost2  InjectionAngPre=MDL.VehicleControl.Miscellaneous.EngineControl.InjectionAngPre  InjectionAngMain=MDL.VehicleControl.Miscellaneous.EngineControl.InjectionAngMain  InjectionAngPost1=MDL.VehicleControl.Miscellaneous.EngineControl.InjectionAngPost1  InjectionAngPost2=MDL.VehicleControl.Miscellaneous.EngineControl.InjectionAngPost2  IntakeCamOffsetAng=MDL.VehicleControl.Miscellaneous.EngineControl.IntakeCamOffsetAng  ExhaustCamOffsetAng=MDL.VehicleControl.Miscellaneous.EngineControl.ExhaustCamOffsetAng  RelativeOpeningEGRValve=MDL.VehicleControl.Miscellaneous.EngineControl.RelativeOpeningEGRValve  Load=MDL.VehicleControl.Miscellaneous.EngineControl.Load
  SuspensionTestRigControl : MiscellaneousControlModules/SuspensionTestRigControl  DATA_NODE=MDL.VehicleControl.Miscellaneous.SuspensionTestRigControl  ClampSwitch=MDL.VehicleControl.Miscellaneous.SuspensionTestRigControl.ClampSwitch
  TemperatureControl : MiscellaneousControlModules/TemperatureControl  DATA_NODE=MDL.VehicleControl.Miscellaneous.TemperatureControl  TransmissionTemp=MDL.VehicleControl.Miscellaneous.TemperatureControl.TransmissionTemp  GearStageTemp=MDL.VehicleControl.Miscellaneous.TemperatureControl.GearStageTemp  TransferCaseTemp=MDL.VehicleControl.Miscellaneous.TemperatureControl.TransferCaseTemp  FrontDifferentialTemp=MDL.VehicleControl.Miscellaneous.TemperatureControl.FrontDifferentialTemp  RearDifferentialTemp=MDL.VehicleControl.Miscellaneous.TemperatureControl.RearDifferentialTemp  RearTransferCaseTemp=MDL.VehicleControl.Miscellaneous.TemperatureControl.RearTransferCaseTemp  Rear2DifferentialTemp=MDL.VehicleControl.Miscellaneous.TemperatureControl.Rear2DifferentialTemp  Rear3DifferentialTemp=MDL.VehicleControl.Miscellaneous.TemperatureControl.Rear3DifferentialTemp  ElecMotorTemp=MDL.VehicleControl.Miscellaneous.TemperatureControl.ElecMotorTemp  GeneratorTemp=MDL.VehicleControl.Miscellaneous.TemperatureControl.GeneratorTemp  CoolantTemp=MDL.VehicleControl.Miscellaneous.TemperatureControl.CoolantTemp
  UserDefinedControl : MiscellaneousControlModules/UserDefinedControl  DATA_NODE=MDL.VehicleControl.Miscellaneous.UserDefinedControl
  UserDefinedControlOutput : Subsystem  Tag=TESIS DYNAware Interface Block  mask{NeedsUpdate=off, SignalInfo=|}
      mask SignalInfo=|
      | {
      |   "Version": "4.6",
      |   "MuxedOutputBusName": "UserDefinedControl",
      |   "MuxedInputBusName": "fromCTRL",
      |   "MuxedInputSelected": false,
      |   "MuxedOutputSelected": true,
      |   "SignalData": [
      |     {
      |       "initialValue": "0.0",
      |       "name": "UserDefined1[-]",
      |       "comment": "User-defined miscellaneous signal 1 (can be edited by the user) ",
      |       "minString": "",
      |       "maxString": "",
      |       "width": 1,
      |       "dataType": 0,
      |       "signalType": 0,
      |       "createSignal": false,
      |       "outputName": "UserDefined1[-]",
      |       "generateSignalAccessBlock": false,
      |       "accessId": "$(parentId).$(blockName).$(outputName)"
      |     },
      |     {
      |       "initialValue": "0.0",
      |       "name": "UserDefined2[-]",
      |       "comment": "User-defined miscellaneous signal 2 (can be edited by the user) ",
      |       "minString": "",
      |       "maxString": "",
      |       "width": 1,
      |       "dataType": 0,
      |       "signalType": 0,
      |       "createSignal": false,
      |       "outputName": "UserDefined2[-]",
      |       "generateSignalAccessBlock": false,
      |       "accessId": "$(parentId).$(blockName).$(outputName)"
      |     }
      |   ]
      | }
      mask prompts: NeedsUpdate "Specify, if subsystem content needs to be updated"; SignalInfo "Signal Info (json)"
      mask help: DYNA4 Interface Block Version 4.6
      mask init:
      | blockName = get_param(gcbh, 'Name');
      | parentId = DYNA4.ModelHandling.AccessID.getFromHierarchy(gcbh);
      | TD.InterfaceBlock.ModelCallbacks.GenerateContent(gcb);
      settings: DeleteFcn=TD.InterfaceBlock.ModelCallbacks.CloseGUI( gcbh );  NameChangeFcn=TD.InterfaceBlock.ModelCallbacks.BlockRenamedHandler(gcbh);  OpenFcn=TD.InterfaceBlock.ModelCallbacks.OpenGUI( gcbh );  CloseFcn=TD.InterfaceBlock.ModelCallbacks.CloseGUI( gcbh );
      mask Display:
      | image('InterfaceBlock.png','center');
      | port_label('input',1, 'UserDefined1[-]');
      | port_label('input',2, 'UserDefined2[-]');
      | port_label('output',1, 'UserDefinedControl');
  BrakeHydraulicsParams : Outport  VectorParamsAs1DForOutWhenUnconnected=off
  EngineControlParams : Outport  Port=2  VectorParamsAs1DForOutWhenUnconnected=off
  SuspensionTestRigControlParams : Outport  Port=3  VectorParamsAs1DForOutWhenUnconnected=off
  TemperatureControlParams : Outport  Port=4  VectorParamsAs1DForOutWhenUnconnected=off
  UserDefinedControlParams : Outport  Port=5  VectorParamsAs1DForOutWhenUnconnected=off
  wires:
  TemperatureControl/1 -> TemperatureControlParams/1
  SuspensionTestRigControl/1 -> SuspensionTestRigControlParams/1
  EngineControl/1 -> EngineControlParams/1
  BrakeHydraulicsControl/1 -> BrakeHydraulicsParams/1
  Abscissae/1 -> BrakeHydraulicsControl/1, SuspensionTestRigControl/1, TemperatureControl/1, UserDefinedControl/1, EngineControl/1
  UserDefinedControlOutput/1(UserDefinedControl___UNIQUE_1) -> UserDefinedControlParams/1
  UserDefinedControl/1 -> Demux/1
  Demux/1 -> UserDefinedControlOutput/1(UserDefined1[-]___UNIQUE_1)
  Demux/2 -> UserDefinedControlOutput/2(UserDefined2[-]___UNIQUE_1)
